simulink model "Closedloop_old"  (R2015b)
settings: Solver=VariableStepAuto  StartTime=0.0  StopTime=100  FixedStep=DT  MaxStep=DT  RelTol=1e-3
values from neighbouring files (symbols this model uses):
  BT = 5    [Run_BorderTest.m]
  Cp = xlsread(filename)    [Run_BorderTest.m]
  Cp_opt = 0.4857    [Run_BorderTest.m]
  lambda_opt = 7.1    [Run_BorderTest.m]
  ng = 87.965    [Run_BorderTest.m]
  R = 35    [Run_BorderTest.m]
  Rho = 1.225    [Run_BorderTest.m]
undefined symbols (not defined in the file or in its folder): OutList, strmatch
settings Model: Creator=bjonkman  LastModifiedBy=alino
settings DataIOCC: SaveFormat=Array  SignalLoggingSaveFormat=ModelDataLogs  SaveOutput=off  SaveTime=off  SignalLoggingName=sigsOut
settings OptimizationCC: ExpressionDepthLimit=2147483647
settings DebuggingCC: SaveWithParameterizedLinksMsg=none  UnderspecifiedInitializationDetection=Classic  MergeDetectMultiDrivingBlocksExec=none  SignalResolutionControl=TryResolveAllWithWarning  MultiTaskDSMMsg=warning  MultiTaskCondExecSysMsg=none  FcnCallInpInsideContextMsg=EnableAllAsWarning  StateNameClashWarn=warning
settings HardwareCC: ProdBitPerPointer=32  ProdLargestAtomicFloat=None  ProdIntDivRoundTo=Undefined  ProdEndianess=Unspecified  ProdWordSize=32  ProdHWDeviceType=32-bit Generic  TargetUnknown=on
settings GRTTargetCC: GeneratePreprocessorConditionals=Disable all  CombineOutputUpdateFcns=off  GRTInterface=on
settings ConfigComp: CovModelRefEnable=Off

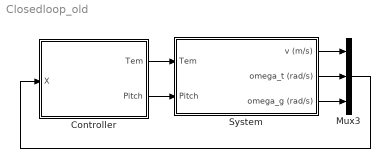
== system Closedloop_old ==
  Controller : Subsystem
  Mux3 : Mux  Inputs=3
  System : Subsystem
  wires:
  Mux3/1 -> Controller/1(X)
  Controller/1("Tem ") -> System/1(Tem)
  Controller/2(Pitch) -> System/2(Pitch)
  System/3(omega_g (rad/s)) -> Mux3/3
  System/2(omega_t (rad/s)) -> Mux3/2
  System/1(v (m/s)) -> Mux3/1

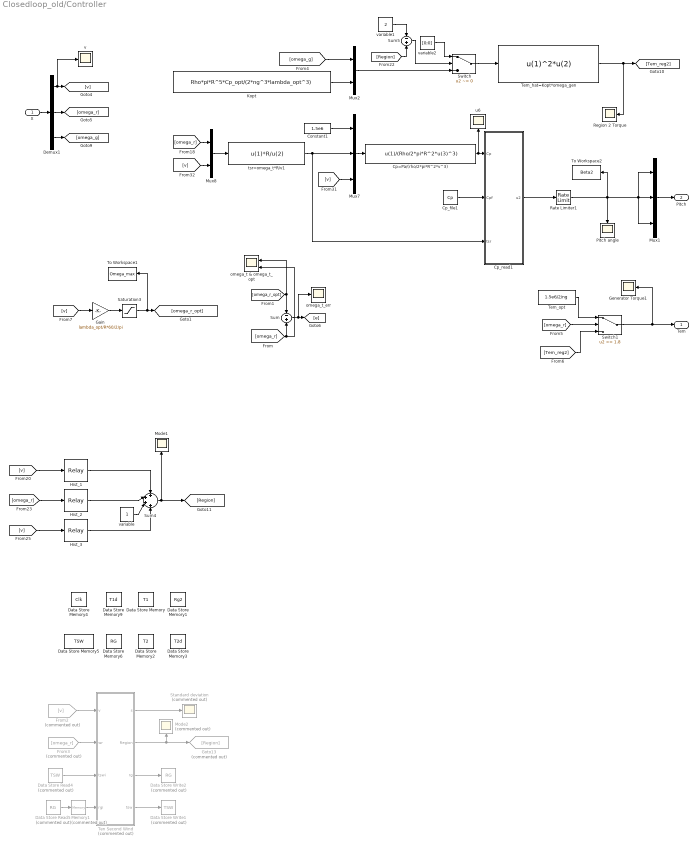
== system Closedloop_old/Controller ==
  X : Inport
  Constant1 : Constant  Value=1.5e6
  Cp=Pa/(rho/2*pi*R^2*v^3) : Fcn  Expr=u(1)/(Rho/2*pi*R^2*u(3)^3)
  Cp_file1 : Constant  Value=Cp
  Cp_read1 : MATLAB Function  TreatAsAtomicUnit=on
  Data Store Memory : DataStoreMemory  DataStoreName=T1
  Data Store Memory1 : DataStoreMemory  DataStoreName=Rg2  InitialValue=1
  Data Store Memory2 : DataStoreMemory  DataStoreName=T2
  Data Store Memory3 : DataStoreMemory  DataStoreName=T2d
  Data Store Memory4 : DataStoreMemory  DataStoreName=Clk
  Data Store Memory5 : DataStoreMemory  DataStoreName=TSW  InitialValue=zeros(1,100)
  Data Store Memory6 : DataStoreMemory  DataStoreName=RG  InitialValue=[0 0 0]  OutDataTypeStr=double
  Data Store Memory9 : DataStoreMemory  DataStoreName=T1d
  Data Store Read4 : DataStoreRead  Commented=on  DataStoreName=TSW
  Data Store Read5 : DataStoreRead  Commented=on  DataStoreName=RG
  Data Store Write1 : DataStoreWrite  Commented=on  DataStoreName=TSW
  Data Store Write2 : DataStoreWrite  Commented=on  DataStoreName=RG
  Demux1 : Demux  Outputs=3
  From2 : From  Commented=on  GotoTag=v
  From3 : From  Commented=on  GotoTag=omega_r
  Gain : Gain  Gain=lambda_opt/R*60/2/pi
  Generator Torque1 : Scope
  Goto13 : Goto  Commented=on  GotoTag=Region
  Hist_1 : Relay  OnSwitchValue=3.3  OffSwitchValue=2.9
  Hist_2 : Relay  OnSwitchValue=1.9  OffSwitchValue=1.8
  Hist_3 : Relay  OnSwitchValue=25  OffSwitchValue=24.8
  "Kopt " : Constant  Value=Rho*pi*R^5*Cp_opt/(2*ng^3*lambda_opt^3)
  Memory1 : Memory  Commented=on
  Mode1 : Scope
  Mode2 : Scope  Commented=on
  Mux1 : Mux  Inputs=3
  Mux2 : Mux  Inputs=2
  Mux7 : Mux  Inputs=3
  Mux8 : Mux  Inputs=2
  Pitch angle : Scope
  Rate Limiter1 : RateLimiter  RisingSlewLimit=5  FallingSlewLimit=-5  SampleTimeMode=inherited
  Region 2 Torque : Scope
  Saturation3 : Saturate  UpperLimit=20.5  LowerLimit=0  ZeroCross=off
  Standard deviation : Scope  Commented=on
  Sum : Sum  Inputs=-+
  Sum4 : Sum  Inputs=++++
  Sum5 : Sum  Inputs=-+
  Switch : Switch  Criteria=u2 ~= 0  Threshold=2
  Switch1 : Switch  Threshold=1.8
  Tem_hat=Kopt*omega_gen : Fcn  Expr=u(1)^2*u(2)
  Tem_opt : Constant  Value=1.5e6/2/ng
  Ten Second Wind : MATLAB Function  Commented=on  TreatAsAtomicUnit=on
  To Workspace1 : ToWorkspace  VariableName=Omega_max  SaveFormat=Timeseries  SampleTime=-1
  To Workspace2 : ToWorkspace  VariableName=Beta2  SaveFormat=Timeseries  SampleTime=-1
  omega_t & omega_t_opt : Scope  NumInputPorts=2
  omega_t_err : Scope
  tsr=omega_t*R/v1 : Fcn  Expr=u(1)*R/u(2)
  u6 : Scope
  v : Scope
  variable : Constant
  variable1 : Constant  Value=2
  variable2 : Constant  Value=[0;0]
  "Tem " : Outport
  Pitch : Outport  Port=2
  wires:
  X/1 -> Demux1/1
  Demux1/1 -> v/1, [v]
  Demux1/2 -> [omega_r]
  Demux1/3 -> [omega_g]
  Sum/1 -> omega_t_err/1, [e]
  [omega_r] -> Sum/2, omega_t & omega_t_opt/2
  [omega_r_opt] -> omega_t & omega_t_opt/1, Sum/1
  Tem_hat=Kopt*omega_gen/1 -> [Tem_reg2], Region 2 Torque/1
  [v] -> Mux7/3
  Mux8/1 -> tsr=omega_t*R/v1/1
  [v] -> Mux8/2
  [omega_r] -> Mux8/1
  tsr=omega_t*R/v1/1 -> Mux7/2, Cp_read1/3(tsr)
  Mux7/1 -> Cp=Pa/(rho/2*pi*R^2*v^3)/1
  Cp=Pa/(rho/2*pi*R^2*v^3)/1 -> u6/1, Cp_read1/1(Cp)
  Cp_file1/1 -> Cp_read1/2(Cpf)
  Constant1/1 -> Mux7/1
  Cp_read1/1(u2) -> Rate Limiter1/1
  Hist_1/1 -> Sum4/1
  [omega_r] -> Hist_2/1
  [v] -> Hist_1/1
  [v] -> Hist_3/1
  Hist_2/1 -> Sum4/2
  Hist_3/1 -> Sum4/4
  variable/1 -> Sum4/3
  Sum4/1 -> [Region], Mode1/1
  [Region] -> Sum5/2
  variable1/1 -> Sum5/1
  Mux1/1 -> Pitch/1
  Sum5/1 -> Switch/2
  variable2/1 -> Switch/1
  Switch/1 -> Tem_hat=Kopt*omega_gen/1
  [omega_g] -> Mux2/1
  "Kopt "/1 -> Mux2/2
  Mux2/1 -> Switch/3
  From2/1 -> Ten Second Wind/1(v)
  Data Store Read4/1 -> Ten Second Wind/3(tswi)
  Ten Second Wind/1(s) -> Standard deviation/1
  Ten Second Wind/2(Region) -> Goto13/1, Mode2/1
  Memory1/1 -> Ten Second Wind/4(rgi)
  Ten Second Wind/4(tsw) -> Data Store Write1/1
  Ten Second Wind/3(rg) -> Data Store Write2/1
  Data Store Read5/1 -> Memory1/1
  From3/1 -> Ten Second Wind/2(wr)
  Switch1/1 -> Generator Torque1/1, "Tem "/1
  Tem_opt/1 -> Switch1/1
  [Tem_reg2] -> Switch1/3
  [omega_r] -> Switch1/2
  [v] -> Gain/1
  Saturation3/1 -> To Workspace1/1, [omega_r_opt]
  Gain/1 -> Saturation3/1
  Rate Limiter1/1 -> To Workspace2/1, Mux1/3, Mux1/2, Mux1/1, Pitch angle/1

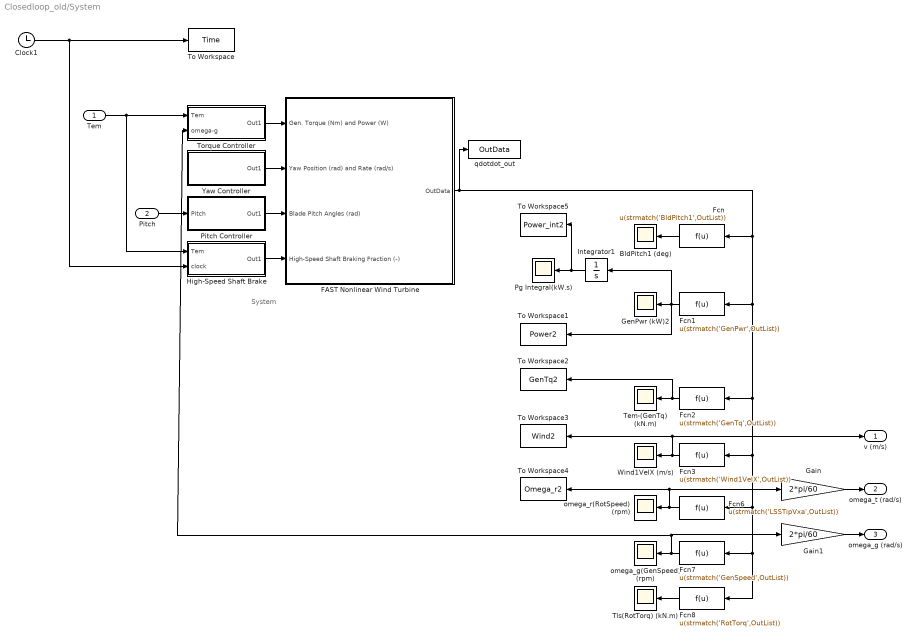
== system Closedloop_old/System ==
  note: System
  Tem : Inport
  Pitch : Inport  Port=2
  BldPitch1 (deg) : Scope
  Clock1 : Clock
  FAST Nonlinear Wind Turbine : Subsystem  mask(FAST Nonlinear Wind Turbine){}
      mask help: This block contains the FAST S-Function.
      mask init:
      | clear FAST_SFunc
  Fcn : Fcn  Expr=u(strmatch('BldPitch1',OutList))
  Fcn1 : Fcn  Expr=u(strmatch('GenPwr',OutList))
  Fcn2 : Fcn  Expr=u(strmatch('GenTq',OutList))
  Fcn3 : Fcn  Expr=u(strmatch('Wind1VelX',OutList))
  Fcn6 : Fcn  Expr=u(strmatch('LSSTipVxa',OutList))
  Fcn7 : Fcn  Expr=u(strmatch('GenSpeed',OutList))
  Fcn8 : Fcn  Expr=u(strmatch('RotTorq',OutList))
  Gain : Gain  Gain=2*pi/60
  Gain1 : Gain  Gain=2*pi/60
  GenPwr (kW)2 : Scope
  High-Speed Shaft Brake : Subsystem
  Integrator1 : Integrator
  Pg Integral(kW.s) : Scope
  Pitch Controller : Subsystem
  Tem-(GenTq) (kN.m) : Scope
  Tls(RotTorq) (kN.m) : Scope
  To Workspace : ToWorkspace  VariableName=Time  SampleTime=-1
  To Workspace1 : ToWorkspace  VariableName=Power2  SaveFormat=Timeseries  SampleTime=-1
  To Workspace2 : ToWorkspace  VariableName=GenTq2  SaveFormat=Timeseries  SampleTime=-1
  To Workspace3 : ToWorkspace  VariableName=Wind2  SaveFormat=Timeseries  SampleTime=-1
  To Workspace4 : ToWorkspace  VariableName=Omega_r2  SaveFormat=Timeseries  SampleTime=-1
  To Workspace5 : ToWorkspace  VariableName=Power_int2  SaveFormat=Timeseries  SampleTime=-1
  Torque Controller : Subsystem
  Wind1VelX (m/s) : Scope
  Yaw Controller : Subsystem
  omega_g(GenSpeed) (rpm) : Scope
  omega_r(RotSpeed) (rpm) : Scope
  qdotdot_out : ToWorkspace  VariableName=OutData  SampleTime=-1
  v (m/s) : Outport
  omega_t (rad/s) : Outport  Port=2
  omega_g (rad/s) : Outport  Port=3
  wires:
  Clock1/1 -> To Workspace/1, High-Speed Shaft Brake/2(clock)
  Torque Controller/1(Out1) -> FAST Nonlinear Wind Turbine/1(Gen. Torque (Nm) and Power (W))
  Yaw Controller/1(Out1) -> FAST Nonlinear Wind Turbine/2(Yaw Position (rad) and Rate (rad/s))
  Pitch Controller/1(Out1) -> FAST Nonlinear Wind Turbine/3(Blade Pitch Angles (rad))
  High-Speed Shaft Brake/1(Out1) -> FAST Nonlinear Wind Turbine/4(High-Speed Shaft Braking Fraction (-))
  Fcn/1 -> BldPitch1 (deg)/1
  Fcn2/1 -> To Workspace2/1, Tem-(GenTq) (kN.m)/1
  Fcn3/1 -> To Workspace3/1, v (m/s)/1, Wind1VelX (m/s)/1
  Fcn6/1 -> To Workspace4/1, Gain/1, omega_r(RotSpeed) (rpm)/1
  Fcn7/1 -> Torque Controller/2(omega-g), Gain1/1, omega_g(GenSpeed) (rpm)/1
  Fcn8/1 -> Tls(RotTorq) (kN.m)/1
  FAST Nonlinear Wind Turbine/1(OutData) -> Fcn8/1, Fcn7/1, Fcn6/1, Fcn3/1, Fcn2/1, Fcn1/1, Fcn/1, qdotdot_out/1
  Tem/1 -> Torque Controller/1(Tem), High-Speed Shaft Brake/1(Tem)
  Gain/1 -> omega_t (rad/s)/1
  Gain1/1 -> omega_g (rad/s)/1
  Pitch/1 -> Pitch Controller/1(Pitch)
  Fcn1/1 -> Integrator1/1, To Workspace1/1, GenPwr (kW)2/1
  Integrator1/1 -> To Workspace5/1, Pg Integral(kW.s)/1

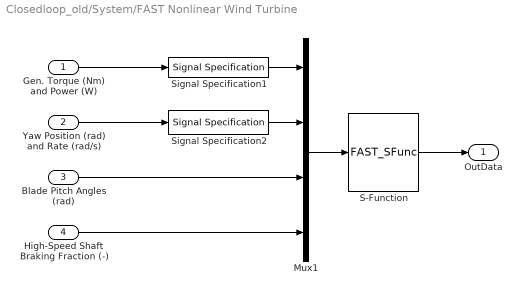
== system Closedloop_old/System/FAST Nonlinear Wind Turbine ==
  Gen. Torque (Nm) and Power (W) : Inport
  Yaw Position (rad) and Rate (rad/s) : Inport  Port=2
  Blade Pitch Angles (rad) : Inport  Port=3
  High-Speed Shaft Braking Fraction (-) : Inport  Port=4
  Mux1 : Mux
  S-Function : S-Function  FunctionName=FAST_SFunc  Parameters=FAST_InputFileName, TMax, 0  SFunctionDeploymentMode=off  EnableBusSupport=off
  Signal Specification1 : SignalSpecification  OutDataTypeStr=double  Dimensions=2
  Signal Specification2 : SignalSpecification  OutDataTypeStr=double  Dimensions=2
  OutData : Outport
  wires:
  Gen. Torque (Nm) and Power (W)/1 -> Signal Specification1/1
  S-Function/1 -> OutData/1
  Mux1/1 -> S-Function/1
  Blade Pitch Angles (rad)/1 -> Mux1/3
  Yaw Position (rad) and Rate (rad/s)/1 -> Signal Specification2/1
  Signal Specification1/1 -> Mux1/1
  Signal Specification2/1 -> Mux1/2
  High-Speed Shaft Braking Fraction (-)/1 -> Mux1/4

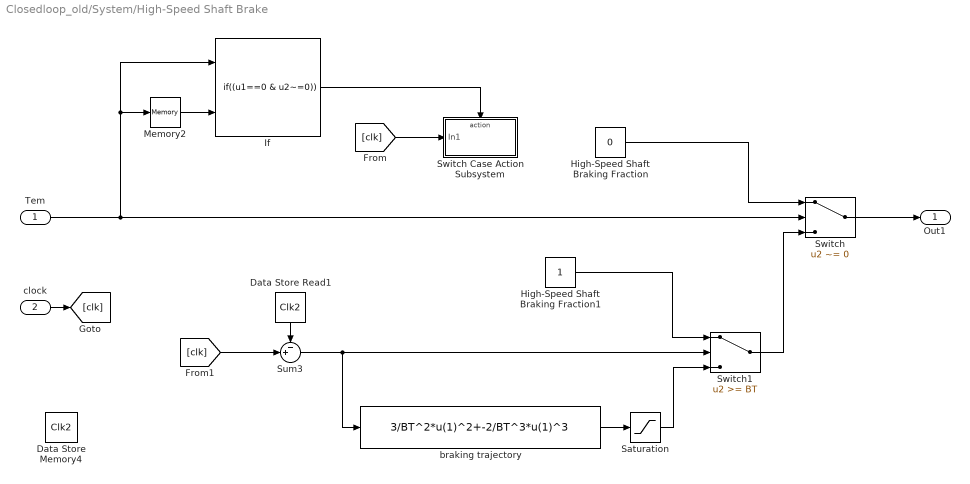
== system Closedloop_old/System/High-Speed Shaft Brake ==
  Tem : Inport
  clock : Inport  Port=2
  Data Store Memory4 : DataStoreMemory  DataStoreName=Clk2
  Data Store Read1 : DataStoreRead  DataStoreName=Clk2  SampleTime=0
  High-Speed Shaft Braking Fraction : Constant  Value=0
  High-Speed Shaft Braking Fraction1 : Constant
  If : If  NumInputs=2  IfExpression=(u1==0 & u2~=0)  ShowElse=off
  Memory2 : Memory
  Saturation : Saturate  UpperLimit=1  LowerLimit=0
  Sum3 : Sum  Inputs=-+|
  Switch : Switch  Criteria=u2 ~= 0
  Switch Case Action Subsystem : Subsystem  TreatAsAtomicUnit=on
  Switch1 : Switch  Threshold=BT  ZeroCross=off
  braking trajectory : Fcn  Expr=3/BT^2*u(1)^2+-2/BT^3*u(1)^3
  Out1 : Outport
  wires:
  Switch/1 -> Out1/1
  High-Speed Shaft Braking Fraction/1 -> Switch/1
  Saturation/1 -> Switch1/3
  If/1 -> Switch Case Action Subsystem/Action
  [clk] -> Switch Case Action Subsystem/1(In1)
  [clk] -> Sum3/2
  Sum3/1 -> Switch1/2, braking trajectory/1
  Data Store Read1/1 -> Sum3/1
  braking trajectory/1 -> Saturation/1
  Memory2/1 -> If/2
  Tem/1 -> If/1, Memory2/1, Switch/2
  Switch1/1 -> Switch/3
  High-Speed Shaft Braking Fraction1/1 -> Switch1/1
  clock/1 -> [clk]

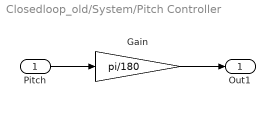
== system Closedloop_old/System/Pitch Controller ==
  Pitch : Inport
  Gain : Gain  Gain=pi/180
  Out1 : Outport
  wires:
  Pitch/1 -> Gain/1
  Gain/1 -> Out1/1

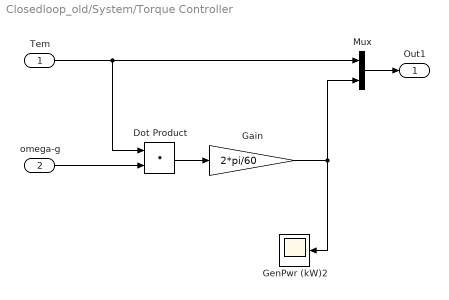
== system Closedloop_old/System/Torque Controller ==
  Tem : Inport
  omega-g : Inport  Port=2
  Dot Product : DotProduct  InputSameDT=on  OutDataTypeStr=Inherit: Inherit via internal rule
  Gain : Gain  Gain=2*pi/60
  GenPwr (kW)2 : Scope
  Mux : Mux  Inputs=2
  Out1 : Outport
  wires:
  Mux/1 -> Out1/1
  Tem/1 -> Dot Product/1, Mux/1
  omega-g/1 -> Dot Product/2
  Dot Product/1 -> Gain/1
  Gain/1 -> GenPwr (kW)2/1, Mux/2

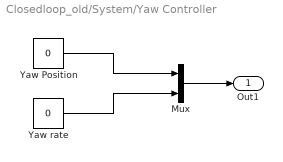
== system Closedloop_old/System/Yaw Controller ==
  Mux : Mux  Inputs=2
  Yaw Position : Constant  Value=0
  Yaw rate : Constant  Value=0
  Out1 : Outport
  wires:
  Mux/1 -> Out1/1
  Yaw Position/1 -> Mux/1
  Yaw rate/1 -> Mux/2

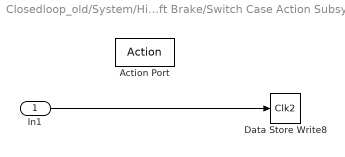
== system Closedloop_old/System/High-Speed Shaft Brake/Switch Case Action Subsystem ==
  In1 : Inport
  Action Port : ActionPort  ActionType=then
  Data Store Write8 : DataStoreWrite  DataStoreName=Clk2
  wires:
  In1/1 -> Data Store Write8/1

== matlab function Closedloop_old/Controller/Cp_read1 ==
  data: Cp input; u2 output; Cpf input; tsr input
function u2 = fcn(Cp,Cpf,tsr)
    tsr=floor(tsr*10+0.5);
    beta=2;
    if (Cp>0) && (Cp<0.4857) && (tsr<200) && (tsr>0)
        i=90;
        while (Cp>Cpf(i,tsr))
            i=i-1;
            if i==2 
                break; 
            end
        end
        if (i>2)
            p=(Cp-Cpf(i+1,tsr))/(Cpf(i,tsr)-Cpf(i+1,tsr));
            beta=(i-p); 
        end
    end
    u2=beta;
end

== matlab function Closedloop_old/Controller/Ten Second Wind ==
  data: v input; wr input; s output; tswi input; Region output; rg output; tsw output; rgi input
function [s,Region,rg,tsw] = fcn(v,wr,tswi,rgi)
    
    tsw=zeros(1,100);
    tsw(1:99)=tswi(2:100);
    tsw(100)=v;
    s=sqrt(var(tsw));
    rg=rgi;
    if v>25
        rg=[1;1;1];
    elseif v<(25-2*s)
        rg(3)=0;
    end
    if wr>(2)
        rg(2)=1;
    elseif wr<(2-2*s)
        rg(2)=0;
    end
    if v>(3+2*s)
        rg(1)=1;
    elseif v<3
        rg=[0;0;0];
    end
    
    Region=rg(1)+rg(2)+rg(3)+1;
end
